simulink model "qn4"  (R2019b)
settings: Solver=VariableStepAuto  StartTime=0.0  StopTime=10.0  RelTol=1e-3
libraries: simulink x1
settings Model: Creator=MHTRON001  LastModifiedBy=MHTRON001

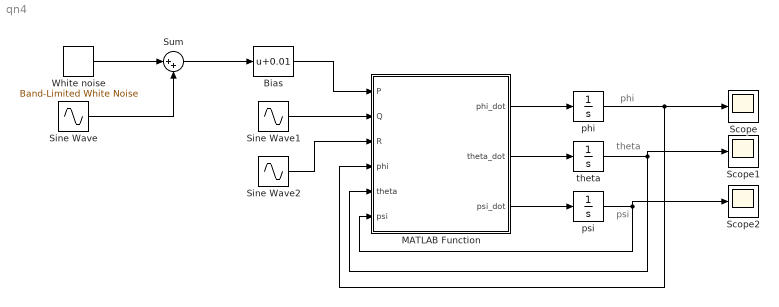
== system qn4 ==
  note: phi
  note: psi
  note: theta
  Bias : Bias  Bias=0.01
  MATLAB Function : MATLAB Function  TreatAsAtomicUnit=on
  Scope : Scope
  Scope1 : Scope
  Scope2 : Scope
  Sine Wave : Sin  SampleTime=0
  Sine Wave1 : Sin  SampleTime=0
  Sine Wave2 : Sin  SampleTime=0
  Sum : Sum  Inputs=|++
  "White noise " : simulink/Sources/Band-Limited White Noise  Cov=0.1*0.02  Ts=0.02  seed=[23242]
  phi : Integrator
  psi : Integrator
  theta : Integrator
  wires:
  MATLAB Function/1(phi_dot) -> phi/1
  MATLAB Function/2(theta_dot) -> theta/1
  MATLAB Function/3(psi_dot) -> psi/1
  phi/1 -> MATLAB Function/4(phi), Scope/1
  theta/1 -> Scope1/1, MATLAB Function/5(theta)
  psi/1 -> Scope2/1, MATLAB Function/6(psi)
  Sine Wave1/1 -> MATLAB Function/2(Q)
  Sine Wave2/1 -> MATLAB Function/3(R)
  "White noise "/1 -> Sum/1
  Sine Wave/1 -> Sum/2
  Sum/1 -> Bias/1
  Bias/1 -> MATLAB Function/1(P)

== matlab function qn4/MATLAB Function ==
  data: P input; Q input; R input; phi_dot output; theta_dot output; psi_dot output; phi input; theta input; psi input
function [phi_dot, theta_dot, psi_dot] = aircraft(P, Q, R, phi, theta, psi)
    
    phi_dot = P + Q*sin(phi)*tan(theta) + R*cos(phi)*tan(theta);
    theta_dot = Q*cos(phi) - R*sin(phi);
    psi_dot = Q*sin(phi)*sec(theta) + R*cos(phi)*sec(theta);
    
end
